simulink model "Controller_testslx"  (R2025a)
settings: Solver=VariableStepAuto  StartTime=0.0  StopTime=0.7  RelTol=1e-3
settings Model: Creator=Eduardoht  LastModifiedBy=Eduardoht

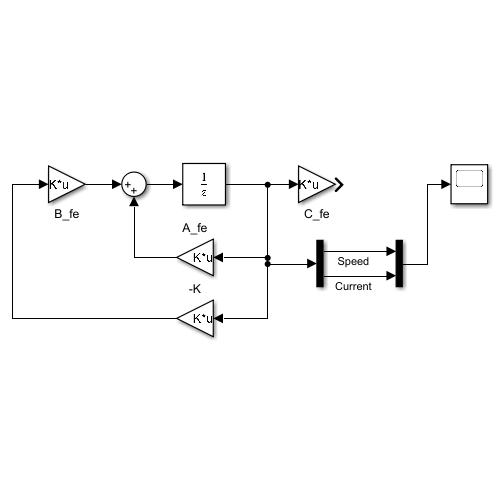
[thumbnail: Simulink's stored preview of the top-level diagram]
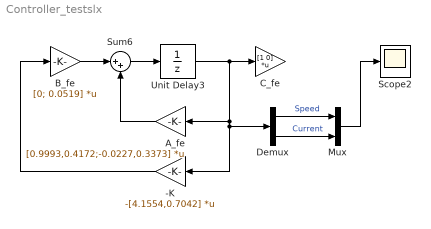
== system Controller_testslx ==
  -K : Gain  Gain=-[4.1554,0.7042]  Multiplication=Matrix(K*u)
  A_fe : Gain  Gain=[0.9993,0.4172;-0.0227,0.3373]  Multiplication=Matrix(K*u)
  B_fe : Gain  Gain=[0; 0.0519]  Multiplication=Matrix(K*u)
  C_fe : Gain  Gain=[1 0]  Multiplication=Matrix(K*u)
  Demux : Demux  Outputs=2
  Mux : Mux  Inputs=2
  Scope2 : Scope
      settings: ActiveDisplayYMinimum=-2.555037284663785  ActiveDisplayYMaximum=6.2991152538515323
  Sum6 : Sum  Inputs=|++
  Unit Delay3 : UnitDelay  InitialCondition=[5; 1];  SampleTime=0.001  HasFrameUpgradeWarning=on
  wires:
  -K/1 -> B_fe/1
  B_fe/1 -> Sum6/1
  A_fe/1 -> Sum6/2
  Sum6/1 -> Unit Delay3/1
  Unit Delay3/1 -> Demux/1, -K/1, A_fe/1, C_fe/1
  Demux/1 -> Mux/1  "Speed"
  Demux/2 -> Mux/2  "Current"
  Mux/1 -> Scope2/1
